simulink model "BMS_BIL_Wrapper"  (R2025b)
settings: Solver=FixedStepAuto  StartTime=0.0  StopTime=10.0  RelTol=1e-3  EnableMultiTasking=on
InitFcn:
  | battery_init;
  | Full_Charge_Volt=4.2; % unit volts
  | Cutoff_Volt=3; % unit volts
  | Delta=.02;
  | ContactorTime=20;
  | ContactorTimeOut=100;
  | High_TempLim=333;
  | Low_TempLim=253;
  | Sensor_Fault_Treshold=.02;
  | CurrentTimeout=1;
  | Allowed_Delta=.04;
  | Bal_On_Time=30;
  | Bal_Off_Time=5;
  | BalNotAct_Time=10;
values from neighbouring files (symbols this model uses):
  ADC_Volt_Resolution = .000089    (= 8.9e-05)    [MCU.m]
  bonka_R0 = [ ... (first row only)    [battery_init.m]
  bonka_SOC = [0, 0.1, 0.2, 0.3, 0.4, 0.5, 0.6, 0.7, 0.8, 0.9, 1.0]    [battery_init.m]
  bonka_T = [263.15, 273.15, 298.15, 313.15, 328.15]    [battery_init.m]
  Capacity = 5.200    (= 5.2)    [MCU.m]
  Charge_Rate = 1    [battery_init.m]
  Discharge_Rate = -1    [battery_init.m]
  R_NTC = 10000    [MCU.m]
  R_Pullup = 10000    [MCU.m]
  R_Sense = .01    (= 0.01)    [MCU.m]
  V_Bat_Div_Res = .00133    (= 0.00133)    [MCU.m]
  V_ISENSE_Res = .00000133    (= 1.33e-06)    [MCU.m]
undefined symbols (not defined in the file or in its folder): DiscIntNeverNeededParam
libraries: simulink x58, stm32f4xxblockslib x1, stm32blockslib x1
(part 1 of 2)
settings Model: DataDictionary=Needed_Buses.sldd  STM32="{\"SPIControllerTransfer\":[{\"ID\":\"Executable_Sim:1\"},{\"ID\":\"BMS_HIL_Wrapper:1\"},{\"ID\":\"BMS_HIL_Wrapper:200\"},{\"ID\":\"BMS_HIL_Wrapper:349\"},{\"ID\":\"BMS_BIL_Wrapper:1\"}],\"DigitalPortWrite\":[{\"ID\":\"Executable_Sim:197\"},{\"ID\":\"Executable_Sim:198\"},{\"ID\":\"BMS_BIL_Wrapper:898\"}]}"  Creator=Odonata-KJ  LastModifiedBy=Odonata-KJ
settings OptimizationCC: DefaultParameterBehavior=Inlined  EnhancedBackFolding=on  PassReuseOutputArgsAs=Individual arguments  ZeroExternalMemoryAtStartup=off  ZeroInternalMemoryAtStartup=off  MaxStackSize=512  OptimizeBlockOrder=speed  DifferentSizesBufferReuse=on  OptimizationCustomize=off  EfficientTunableParamExpr=on
settings DebuggingCC: ParameterTunabilityLossMsg=error
settings HardwareCC: ProdBitPerPointer=32.0  ProdBitPerSizeT=32.0  ProdBitPerPtrDiffT=32.0  ProdLargestAtomicInteger=Long  ProdLargestAtomicFloat=Double  ProdWordSize=32.0  ProdLongLongMode=on  ProdHWDeviceType=ARM Compatible->ARM Cortex-M  TargetBitPerPointer=64.0  TargetBitPerSizeT=64.0  TargetBitPerPtrDiffT=64.0  TargetLongLongMode=on  TargetIntDivRoundTo=Zero  TargetEndianess=LittleEndian  TargetWordSize=64.0  TargetHWDeviceType=MATLAB Host  ProdEqTarget=off
settings SFSimCC: MATLABDynamicMemAlloc=off
settings RTWCC: SystemTargetFile=ert.tlc  HardwareBoard=STM32F4xx Based  TemplateMakefile=ert_default_tmf  Toolchain=GNU Tools for ARM Embedded Processors  BuildConfiguration=Faster Runs  Description=Embedded Coder
settings CodeAppCC: ForceParamTrailComments=on  IgnoreCustomStorageClasses=off  OperatorAnnotations=on  SimulinkDataObjDesc=on  SFDataObjDesc=on  InsertBlockDesc=on
settings ERTTargetCC: ExtModeTransport=3.0  ExtModeStaticAlloc=on  ExtModeStaticAllocSize=2048.0  ExtModeMexFile=ext_xcp  ExtModeIntrfLevel=Level2 - Open  TargetLangStandard=C99 (ISO)

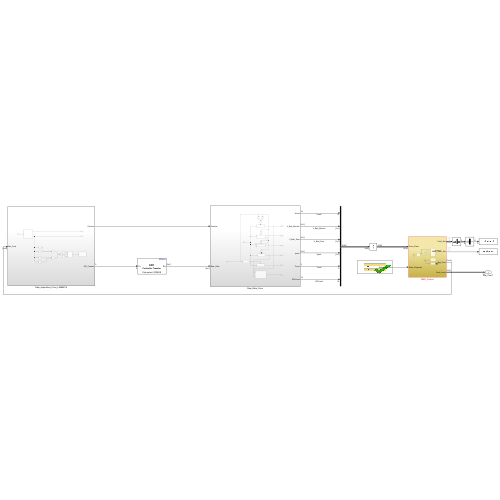
[thumbnail: Simulink's stored preview of the top-level diagram]
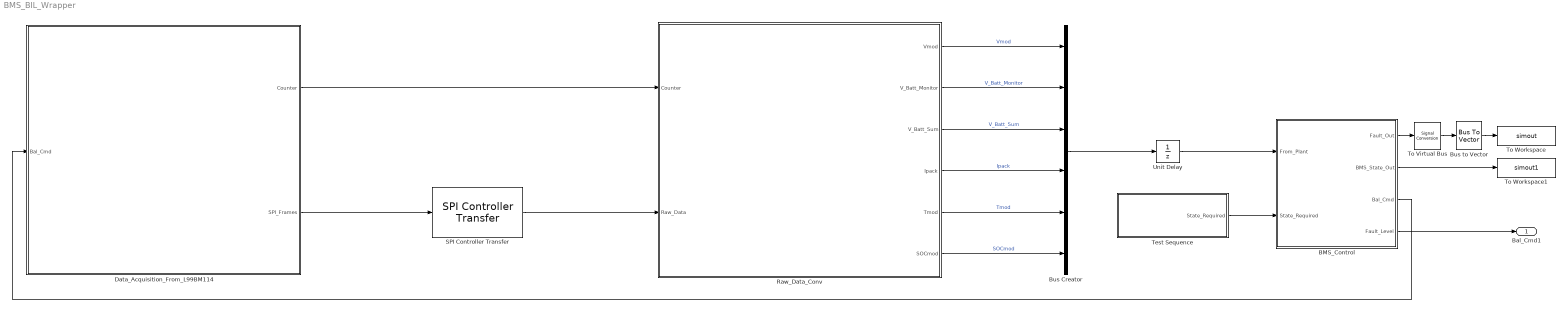
== system BMS_BIL_Wrapper ==
  BMS_Control : Subsystem
  Bus Creator : BusCreator  Inputs=6
  Bus to Vector : BusToVector
  Data_Acquisition_From_L99BM114 : Subsystem
  Raw_Data_Conv : Subsystem
  SPI Controller Transfer : stm32blockslib/SPI Controller Transfer  SPIModuleSelect=SPI1  ClockPolarity=Low  ClockPhase=1 Edge  SPIModule=uint32(0)  Mode=Master  BusSpeed=uint32(1000000)  FirstBitToTransfer=Most significant bit (MSB)  ClockMode=0  BlockFunction=Transfer  EnableRegisterAddress=on  RegisterAddress=0  OutputDataType=uint8  OutputDataLength=1  OutputStatus=off  BlockingMode=off  Timeout=0.001  DataBits=8  UseCustomSSPin=Provided by the SPI peripheral  ActiveLowSSPin=Active low  Port_Select=GPIOA  Pin=0
      settings: LibrarySourceBlock=stm32f4xxblockslib/SPI Controller Transfer
  Test Sequence : Test Sequence  TreatAsAtomicUnit=on
  To Virtual Bus : SignalConversion  ConversionOutput=Virtual bus  OverrideOpt=off
  To Workspace : ToWorkspace  VariableName=simout  SaveFormat=Structure With Time  SampleTime=-1
  To Workspace1 : ToWorkspace  VariableName=simout1  SaveFormat=Structure With Time  SampleTime=-1
  Unit Delay : UnitDelay  SampleTime=-1  HasFrameUpgradeWarning=on
  Bal_Cmd1 : Outport
  wires:
  Bus Creator/1 -> Unit Delay/1
  Test Sequence/1(State_Required) -> BMS_Control/2(State_Required)
  BMS_Control/1(Fault_Out) -> To Virtual Bus/1
  Data_Acquisition_From_L99BM114/2(SPI_Frames) -> SPI Controller Transfer/1
  SPI Controller Transfer/1 -> Raw_Data_Conv/2(Raw_Data)
  Raw_Data_Conv/1(Vmod) -> Bus Creator/1  "Vmod"
  Raw_Data_Conv/2(V_Batt_Monitor) -> Bus Creator/2  "V_Batt_Monitor"
  Raw_Data_Conv/3(V_Batt_Sum) -> Bus Creator/3  "V_Batt_Sum"
  Raw_Data_Conv/4(Ipack) -> Bus Creator/4  "Ipack"
  Raw_Data_Conv/5(Tmod) -> Bus Creator/5  "Tmod"
  Raw_Data_Conv/6(SOCmod) -> Bus Creator/6  "SOCmod"
  Data_Acquisition_From_L99BM114/1(Counter) -> Raw_Data_Conv/1(Counter)
  BMS_Control/2(BMS_State_Out) -> To Workspace1/1
  Bus to Vector/1 -> To Workspace/1
  To Virtual Bus/1 -> Bus to Vector/1
  BMS_Control/4(Fault_Level) -> Bal_Cmd1/1
  BMS_Control/3(Bal_Cmd) -> Data_Acquisition_From_L99BM114/1(Bal_Cmd)
  Unit Delay/1 -> BMS_Control/1(From_Plant)

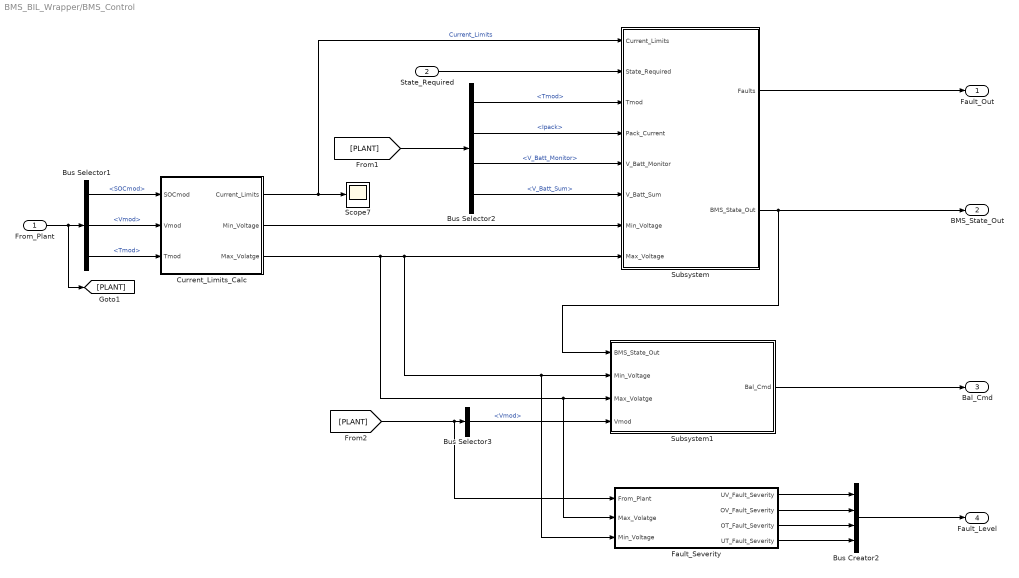
== system BMS_BIL_Wrapper/BMS_Control ==
  From_Plant : Inport
  State_Required : Inport  Port=2
  Bus Creator2 : BusCreator  Inputs=4
  Bus Selector1 : BusSelector  OutputSignals=SOCmod,Vmod,Tmod
  Bus Selector2 : BusSelector  OutputSignals=Tmod,Ipack,V_Batt_Monitor,V_Batt_Sum
  Bus Selector3 : BusSelector  OutputSignals=Vmod
  Current_Limits_Calc : Subsystem
  Fault_Severity : Subsystem
  Scope7 : Scope
      settings: ActiveDisplayYMinimum=-204.94239490667829  ActiveDisplayYMaximum=69.203108892530651  DataLoggingVariableName=ScopeData14
  Subsystem : Subsystem
  Subsystem1 : Subsystem
  Fault_Out : Outport
  BMS_State_Out : Outport  Port=2
  Bal_Cmd : Outport  Port=3
  Fault_Level : Outport  Port=4
  wires:
  Subsystem/2(BMS_State_Out) -> Subsystem1/1(BMS_State_Out), BMS_State_Out/1
  Subsystem/1(Faults) -> Fault_Out/1
  [PLANT] -> Bus Selector2/1
  State_Required/1 -> Subsystem/2(State_Required)
  Current_Limits_Calc/1(Current_Limits) -> Scope7/1, Subsystem/1(Current_Limits)  "Current_Limits"
  Current_Limits_Calc/3(Max_Volatge) -> Fault_Severity/2(Max_Volatge), Subsystem1/3(Max_Volatge), Fault_Severity/3(Min_Voltage), Subsystem1/2(Min_Voltage), Subsystem/8(Max_Voltage)
  Current_Limits_Calc/2(Min_Voltage) -> Subsystem/7(Min_Voltage)
  From_Plant/1 -> Bus Selector1/1, [PLANT]
  Bus Selector2/1 -> Subsystem/3(Tmod)  "<Tmod>"
  Bus Selector2/3 -> Subsystem/5(V_Batt_Monitor)  "<V_Batt_Monitor>"
  Bus Selector2/4 -> Subsystem/6(V_Batt_Sum)  "<V_Batt_Sum>"
  Bus Selector1/1 -> Current_Limits_Calc/1(SOCmod)  "<SOCmod>"
  Bus Selector1/2 -> Current_Limits_Calc/2(Vmod)  "<Vmod>"
  Bus Selector1/3 -> Current_Limits_Calc/3(Tmod)  "<Tmod>"
  Bus Selector2/2 -> Subsystem/4(Pack_Current)  "<Ipack>"
  Fault_Severity/4(UT_Fault_Severity) -> Bus Creator2/4
  Fault_Severity/1(UV_Fault_Severity) -> Bus Creator2/1
  Fault_Severity/2(OV_Fault_Severity) -> Bus Creator2/2
  Fault_Severity/3(OT_Fault_Severity) -> Bus Creator2/3
  [PLANT] -> Fault_Severity/1(From_Plant), Bus Selector3/1
  Bus Selector3/1 -> Subsystem1/4(Vmod)  "<Vmod>"
  Subsystem1/1(Bal_Cmd) -> Bal_Cmd/1
  Bus Creator2/1 -> Fault_Level/1

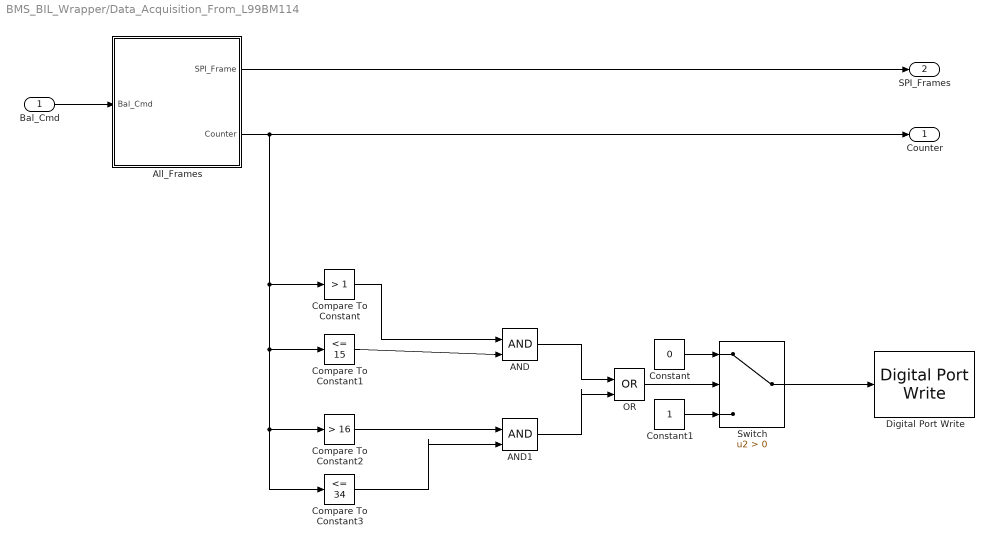
== system BMS_BIL_Wrapper/Data_Acquisition_From_L99BM114 ==
  Bal_Cmd : Inport
  AND : Logic  IconShape=distinctive  AllPortsSameDT=off  OutDataTypeStr=boolean
  AND1 : Logic  IconShape=distinctive  AllPortsSameDT=off  OutDataTypeStr=boolean
  All_Frames : Subsystem
  Compare To Constant : simulink/Logic and Bit Operations/Compare To Constant  relop=>  const=1  OutDataTypeStr=boolean
  Compare To Constant1 : simulink/Logic and Bit Operations/Compare To Constant  relop=<=  const=15  OutDataTypeStr=boolean
  Compare To Constant2 : simulink/Logic and Bit Operations/Compare To Constant  relop=>  const=16  OutDataTypeStr=boolean
  Compare To Constant3 : simulink/Logic and Bit Operations/Compare To Constant  relop=<=  const=34  OutDataTypeStr=boolean
  Constant : Constant  Value=0
  Constant1 : Constant
  Digital Port Write : stm32f4xxblockslib/Digital Port Write  PortName=GPIOB  PinNumber=[0]  ReadOperation=off  IOAsArray=on  EnableSimPort=off  hoistedMaskSrc=ECSoC/ECSimCodegen/Digital Port Write
  OR : Logic  Operator=OR  IconShape=distinctive  AllPortsSameDT=off  OutDataTypeStr=boolean
  Switch : Switch  Criteria=u2 > Threshold  SaturateOnIntegerOverflow=off  InputSameDT=off
  Counter : Outport
  SPI_Frames : Outport  Port=2
  wires:
  All_Frames/2(Counter) -> Compare To Constant2/1, Compare To Constant3/1, Compare To Constant1/1, Compare To Constant/1, Counter/1
  All_Frames/1(SPI_Frame) -> SPI_Frames/1
  Bal_Cmd/1 -> All_Frames/1(Bal_Cmd)
  Compare To Constant/1 -> AND/1
  Compare To Constant1/1 -> AND/2
  AND/1 -> OR/1
  Compare To Constant2/1 -> AND1/1
  Compare To Constant3/1 -> AND1/2
  AND1/1 -> OR/2
  OR/1 -> Switch/2
  Constant/1 -> Switch/1
  Constant1/1 -> Switch/3
  Switch/1 -> Digital Port Write/1

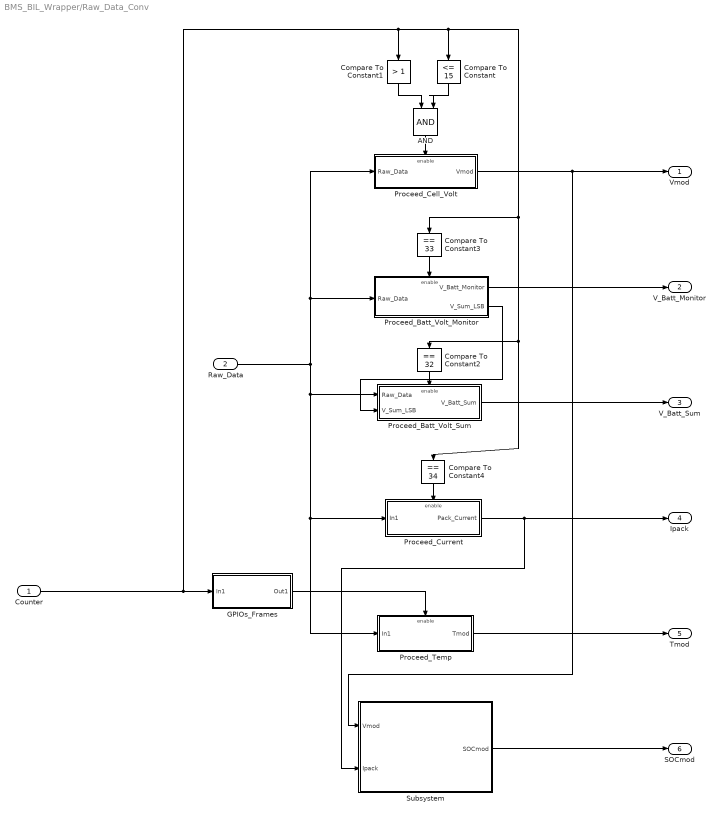
== system BMS_BIL_Wrapper/Raw_Data_Conv ==
  Counter : Inport
  Raw_Data : Inport  Port=2
  AND : Logic  IconShape=distinctive  AllPortsSameDT=off  OutDataTypeStr=boolean
  Compare To Constant : simulink/Logic and Bit Operations/Compare To Constant  relop=<=  const=15  OutDataTypeStr=boolean
  Compare To Constant1 : simulink/Logic and Bit Operations/Compare To Constant  relop=>  const=1  OutDataTypeStr=boolean
  Compare To Constant2 : simulink/Logic and Bit Operations/Compare To Constant  relop===  const=32  OutDataTypeStr=boolean
  Compare To Constant3 : simulink/Logic and Bit Operations/Compare To Constant  relop===  const=33  OutDataTypeStr=boolean
  Compare To Constant4 : simulink/Logic and Bit Operations/Compare To Constant  relop===  const=34  OutDataTypeStr=boolean
  GPIOs_Frames : Subsystem
  Proceed_Batt_Volt_Monitor : Subsystem  TreatAsAtomicUnit=on
  Proceed_Batt_Volt_Sum : Subsystem  TreatAsAtomicUnit=on
  Proceed_Cell_Volt : Subsystem  TreatAsAtomicUnit=on
  Proceed_Current : Subsystem
  Proceed_Temp : Subsystem
  Subsystem : Subsystem
  Vmod : Outport
  V_Batt_Monitor : Outport  Port=2
  V_Batt_Sum : Outport  Port=3
  Ipack : Outport  Port=4
  Tmod : Outport  Port=5
  SOCmod : Outport  Port=6
  wires:
  Proceed_Current/1(Pack_Current) -> Ipack/1, Subsystem/2(Ipack)
  Raw_Data/1 -> Proceed_Cell_Volt/1(Raw_Data), Proceed_Batt_Volt_Monitor/1(Raw_Data), Proceed_Temp/1(In1), Proceed_Current/1(In1), Proceed_Batt_Volt_Sum/1(Raw_Data)
  AND/1 -> Proceed_Cell_Volt/Enable
  Proceed_Batt_Volt_Monitor/2(V_Sum_LSB) -> Proceed_Batt_Volt_Sum/2(V_Sum_LSB)
  Proceed_Batt_Volt_Sum/1(V_Batt_Sum) -> V_Batt_Sum/1
  GPIOs_Frames/1(Out1) -> Proceed_Temp/Enable
  Counter/1 -> Compare To Constant3/1, Compare To Constant2/1, Compare To Constant4/1, Compare To Constant/1, Compare To Constant1/1, GPIOs_Frames/1(In1)
  Compare To Constant2/1 -> Proceed_Batt_Volt_Sum/Enable
  Compare To Constant1/1 -> AND/1
  Compare To Constant/1 -> AND/2
  Compare To Constant3/1 -> Proceed_Batt_Volt_Monitor/Enable
  Compare To Constant4/1 -> Proceed_Current/Enable
  Proceed_Temp/1(Tmod) -> Tmod/1
  Proceed_Cell_Volt/1(Vmod) -> Vmod/1, Subsystem/1(Vmod)
  Subsystem/1(SOCmod) -> SOCmod/1
  Proceed_Batt_Volt_Monitor/1(V_Batt_Monitor) -> V_Batt_Monitor/1

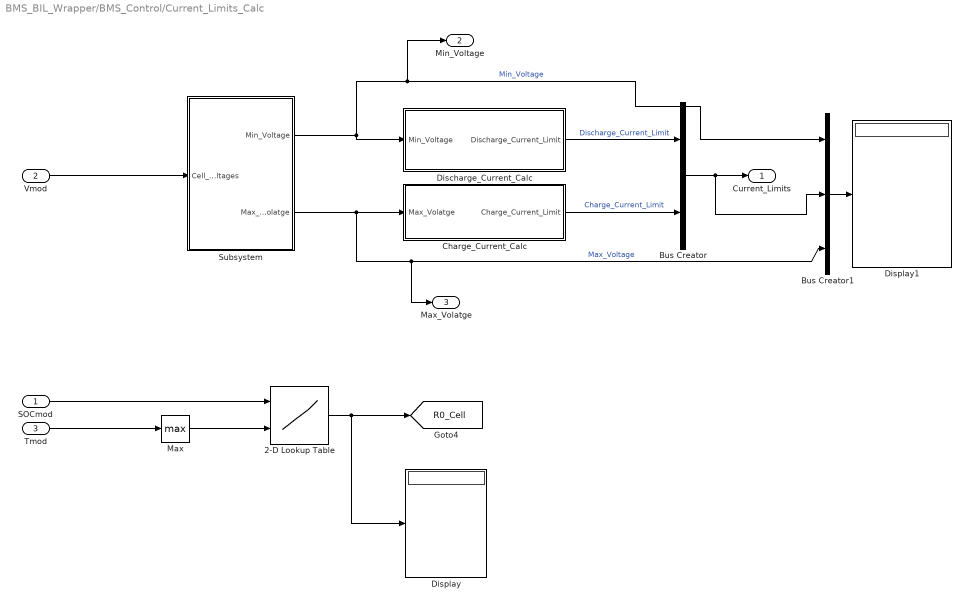
== system BMS_BIL_Wrapper/BMS_Control/Current_Limits_Calc ==
  SOCmod : Inport
  Vmod : Inport  Port=2
  Tmod : Inport  Port=3
  2-D Lookup Table : Lookup_n-D  BreakpointsForDimension1=bonka_SOC  BreakpointsForDimension2=bonka_T  Table=bonka_R0  InternalRulePriority=Speed  RndMeth=Simplest
      settings: InputPortMap=u0,u1
  Bus Creator : BusCreator  Inputs=2
  Bus Creator1 : BusCreator  Inputs=3
  Charge_Current_Calc : Subsystem
  Discharge_Current_Calc : Subsystem
  Display : Display
  Display1 : Display
  Max : MinMax  Function=max
  Subsystem : Subsystem
  Current_Limits : Outport
  Min_Voltage : Outport  Port=2
  Max_Volatge : Outport  Port=3
  tag scope: R0_Cell=global
  wires:
  Max/1 -> 2-D Lookup Table/2
  2-D Lookup Table/1 -> [R0_Cell], Display/1
  SOCmod/1 -> 2-D Lookup Table/1
  Bus Creator1/1 -> Display1/1
  Bus Creator/1 -> Current_Limits/1, Bus Creator1/2
  Charge_Current_Calc/1(Charge_Current_Limit) -> Bus Creator/2  "Charge_Current_Limit"
  Discharge_Current_Calc/1(Discharge_Current_Limit) -> Bus Creator/1  "Discharge_Current_Limit"
  Subsystem/2(Max_Volatge) -> Charge_Current_Calc/1(Max_Volatge), Max_Volatge/1, Bus Creator1/3  "Max_Voltage"
  Tmod/1 -> Max/1
  Subsystem/1(Min_Voltage) -> Min_Voltage/1, Bus Creator1/1, Discharge_Current_Calc/1(Min_Voltage)  "Min_Voltage"
  Vmod/1 -> Subsystem/1(Cell_Voltages)

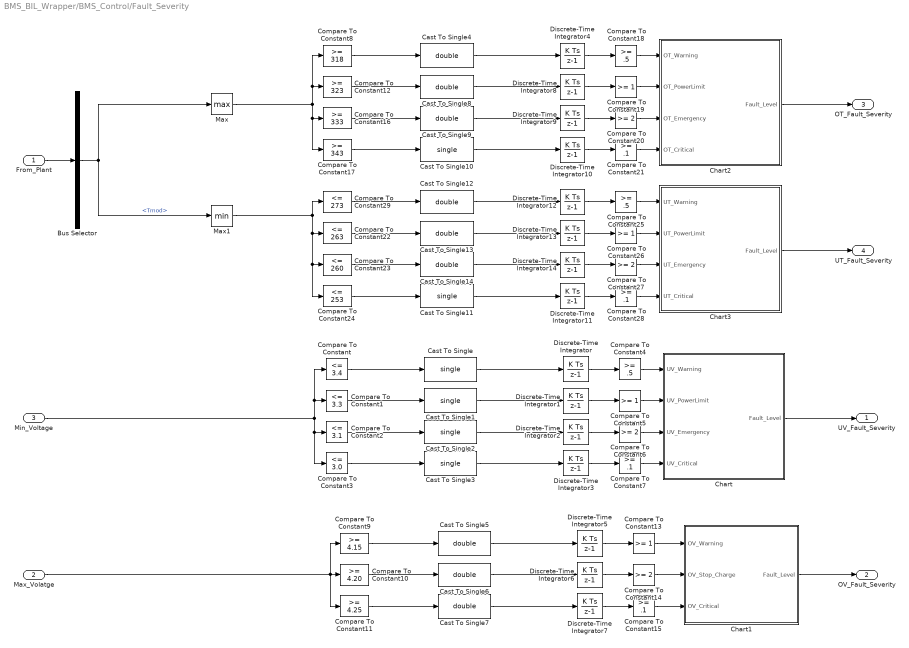
== system BMS_BIL_Wrapper/BMS_Control/Fault_Severity ==
  From_Plant : Inport
  Max_Volatge : Inport  Port=2
  Min_Voltage : Inport  Port=3
  Bus Selector : BusSelector  OutputSignals=Tmod
  Cast To Single{,1..3,10..11} (6 alike) : DataTypeConversion  OutDataTypeStr=single  SaturateOnIntegerOverflow=off  RndMeth=Floor
  Cast To Single{4..9,12..14} (9 alike) : DataTypeConversion  OutDataTypeStr=double  SaturateOnIntegerOverflow=off  RndMeth=Floor
  Chart : Stateflow chart  TreatAsAtomicUnit=on
  Chart1 : Stateflow chart  TreatAsAtomicUnit=on
  Chart2 : Stateflow chart  TreatAsAtomicUnit=on
  Chart3 : Stateflow chart  TreatAsAtomicUnit=on
  Compare To Constant : simulink/Logic and Bit Operations/Compare To Constant  relop=<=  const=3.4  OutDataTypeStr=boolean
  Compare To Constant1 : simulink/Logic and Bit Operations/Compare To Constant  relop=<=  const=3.3  OutDataTypeStr=boolean
  Compare To Constant10 : simulink/Logic and Bit Operations/Compare To Constant  relop=>=  const=4.20  OutDataTypeStr=boolean
  Compare To Constant11 : simulink/Logic and Bit Operations/Compare To Constant  relop=>=  const=4.25  OutDataTypeStr=boolean
  Compare To Constant12 : simulink/Logic and Bit Operations/Compare To Constant  relop=>=  const=323  OutDataTypeStr=boolean
  Compare To Constant{5,13,19,26} (4 alike) : simulink/Logic and Bit Operations/Compare To Constant  relop=>=  const=1  OutDataTypeStr=boolean
  Compare To Constant{6,14,20,27} (4 alike) : simulink/Logic and Bit Operations/Compare To Constant  relop=>=  const=2  OutDataTypeStr=boolean
  Compare To Constant{7,15,21,28} (4 alike) : simulink/Logic and Bit Operations/Compare To Constant  relop=>=  const=.1  OutDataTypeStr=boolean
  Compare To Constant16 : simulink/Logic and Bit Operations/Compare To Constant  relop=>=  const=333  OutDataTypeStr=boolean
  Compare To Constant17 : simulink/Logic and Bit Operations/Compare To Constant  relop=>=  const=343  OutDataTypeStr=boolean
  Compare To Constant18 : simulink/Logic and Bit Operations/Compare To Constant  relop=>=  const=.5  OutDataTypeStr=boolean
  Compare To Constant2 : simulink/Logic and Bit Operations/Compare To Constant  relop=<=  const=3.1  OutDataTypeStr=boolean
  Compare To Constant22 : simulink/Logic and Bit Operations/Compare To Constant  relop=<=  const=263  OutDataTypeStr=boolean
  Compare To Constant23 : simulink/Logic and Bit Operations/Compare To Constant  relop=<=  const=260  OutDataTypeStr=boolean
  Compare To Constant24 : simulink/Logic and Bit Operations/Compare To Constant  relop=<=  const=253  OutDataTypeStr=boolean
  Compare To Constant25 : simulink/Logic and Bit Operations/Compare To Constant  relop=>=  const=.5  OutDataTypeStr=boolean
  Compare To Constant29 : simulink/Logic and Bit Operations/Compare To Constant  relop=<=  const=273  OutDataTypeStr=boolean
  Compare To Constant3 : simulink/Logic and Bit Operations/Compare To Constant  relop=<=  const=3.0  OutDataTypeStr=boolean
  Compare To Constant4 : simulink/Logic and Bit Operations/Compare To Constant  relop=>=  const=.5  OutDataTypeStr=boolean
  Compare To Constant8 : simulink/Logic and Bit Operations/Compare To Constant  relop=>=  const=318  OutDataTypeStr=boolean
  Compare To Constant9 : simulink/Logic and Bit Operations/Compare To Constant  relop=>=  const=4.15  OutDataTypeStr=boolean
  Discrete-Time Integrator{,1..14} (15 alike) : DiscreteIntegrator  SampleTime=.001  ICPrevOutput=DiscIntNeverNeededParam  ICPrevScaledInput=DiscIntNeverNeededParam
  Max : MinMax  Function=max
  Max1 : MinMax
  UV_Fault_Severity : Outport
  OV_Fault_Severity : Outport  Port=2
  OT_Fault_Severity : Outport  Port=3
  UT_Fault_Severity : Outport  Port=4
  wires:
  From_Plant/1 -> Bus Selector/1
  Min_Voltage/1 -> Compare To Constant3/1, Compare To Constant2/1, Compare To Constant/1, Compare To Constant1/1
  Compare To Constant/1 -> Cast To Single/1
  Compare To Constant1/1 -> Cast To Single1/1
  Compare To Constant2/1 -> Cast To Single2/1
  Compare To Constant3/1 -> Cast To Single3/1
  Cast To Single/1 -> Discrete-Time Integrator/1
  Cast To Single1/1 -> Discrete-Time Integrator1/1
  Cast To Single2/1 -> Discrete-Time Integrator2/1
  Discrete-Time Integrator/1 -> Compare To Constant4/1
  Discrete-Time Integrator1/1 -> Compare To Constant5/1
  Discrete-Time Integrator2/1 -> Compare To Constant6/1
  Discrete-Time Integrator3/1 -> Compare To Constant7/1
  Cast To Single3/1 -> Discrete-Time Integrator3/1
  Compare To Constant4/1 -> Chart/1(UV_Warning)
  Compare To Constant5/1 -> Chart/2(UV_PowerLimit)
  Compare To Constant6/1 -> Chart/3(UV_Emergency)
  Compare To Constant7/1 -> Chart/4(UV_Critical)
  Chart/1(Fault_Level) -> UV_Fault_Severity/1
  Compare To Constant14/1 -> Chart1/2(OV_Stop_Charge)
  Max_Volatge/1 -> Compare To Constant9/1, Compare To Constant11/1, Compare To Constant10/1
  Discrete-Time Integrator6/1 -> Compare To Constant14/1
  Discrete-Time Integrator5/1 -> Compare To Constant13/1
  Compare To Constant13/1 -> Chart1/1(OV_Warning)
  Cast To Single6/1 -> Discrete-Time Integrator6/1
  Cast To Single7/1 -> Discrete-Time Integrator7/1
  Compare To Constant10/1 -> Cast To Single6/1
  Compare To Constant9/1 -> Cast To Single5/1
  Compare To Constant15/1 -> Chart1/3(OV_Critical)
  Compare To Constant11/1 -> Cast To Single7/1
  Chart1/1(Fault_Level) -> OV_Fault_Severity/1
  Discrete-Time Integrator7/1 -> Compare To Constant15/1
  Cast To Single5/1 -> Discrete-Time Integrator5/1
  Bus Selector/1 -> Max/1, Max1/1  "<Tmod>"
  Discrete-Time Integrator4/1 -> Compare To Constant18/1
  Compare To Constant20/1 -> Chart2/3(OT_Emergency)
  Max/1 -> Compare To Constant8/1, Compare To Constant12/1, Compare To Constant17/1, Compare To Constant16/1
  Discrete-Time Integrator9/1 -> Compare To Constant20/1
  Discrete-Time Integrator8/1 -> Compare To Constant19/1
  Compare To Constant19/1 -> Chart2/2(OT_PowerLimit)
  Cast To Single9/1 -> Discrete-Time Integrator9/1
  Cast To Single10/1 -> Discrete-Time Integrator10/1
  Cast To Single4/1 -> Discrete-Time Integrator4/1
  Compare To Constant16/1 -> Cast To Single9/1
  Compare To Constant12/1 -> Cast To Single8/1
  Compare To Constant21/1 -> Chart2/4(OT_Critical)
  Compare To Constant8/1 -> Cast To Single4/1
  Compare To Constant18/1 -> Chart2/1(OT_Warning)
  Compare To Constant17/1 -> Cast To Single10/1
  Chart2/1(Fault_Level) -> OT_Fault_Severity/1
  Discrete-Time Integrator10/1 -> Compare To Constant21/1
  Cast To Single8/1 -> Discrete-Time Integrator8/1
  Compare To Constant25/1 -> Chart3/1(UT_Warning)
  Max1/1 -> Compare To Constant22/1, Compare To Constant23/1, Compare To Constant24/1, Compare To Constant29/1
  Chart3/1(Fault_Level) -> UT_Fault_Severity/1
  Compare To Constant24/1 -> Cast To Single11/1
  Compare To Constant22/1 -> Cast To Single13/1
  Cast To Single13/1 -> Discrete-Time Integrator13/1
  Compare To Constant29/1 -> Cast To Single12/1
  Discrete-Time Integrator11/1 -> Compare To Constant28/1
  Compare To Constant23/1 -> Cast To Single14/1
  Discrete-Time Integrator14/1 -> Compare To Constant27/1
  Cast To Single14/1 -> Discrete-Time Integrator14/1
  Compare To Constant26/1 -> Chart3/2(UT_PowerLimit)
  Compare To Constant28/1 -> Chart3/4(UT_Critical)
  Cast To Single12/1 -> Discrete-Time Integrator12/1
  Discrete-Time Integrator13/1 -> Compare To Constant26/1
  Discrete-Time Integrator12/1 -> Compare To Constant25/1
  Compare To Constant27/1 -> Chart3/3(UT_Emergency)
  Cast To Single11/1 -> Discrete-Time Integrator11/1

== system BMS_BIL_Wrapper/BMS_Control/Subsystem ==
  Current_Limits : Inport
  State_Required : Inport  Port=2
  Tmod : Inport  Port=3
  Pack_Current : Inport  Port=4  OutDataTypeStr=single
  V_Batt_Monitor : Inport  Port=5
  V_Batt_Sum : Inport  Port=6  OutDataTypeStr=single
  Min_Voltage : Inport  Port=7
  Max_Voltage : Inport  Port=8
  BMS_States : Stateflow chart  TreatAsAtomicUnit=on
      settings: PortSchema="{\"entries\":[{\"content\":{\"sides\":[{\"content\":{\"connectorIds\":[\"In1\",\"In5\",\"In2\",\"In3\",\"In6\",\"In7\",\"In4\",\"In8\"]},\"type\":\"ConnectorPlacement.EquallySpacedRectSide\",\"uuid\":\"75752650-a65f-4df2-8429-36d8f2b8ac99\"},{\"content\":{\"connectorIds\":[\"Out1\",\"Out2\"],\"side\":\"RIGHT\"},\"type\":\"ConnectorPlacement.EquallySpacedRectSide\",\"uuid\":\"5c64a1aa-fdb2-4c0c-b2ff-5c47ddc01ea2\"},{\"content\":{\"side\":\"TOP\"},\"type\":\"ConnectorPlacement.EquallySpacedRectSide\",\"uuid\":\"c92e07e0-a1c3-44d4-87a0-5a0cb4ce56f3\"}]},\"type\":\"ConnectorPlacement.EquallySpacedConnector\",\"uuid\":\"9d97857d-a16c-4ff3-995b-4c10703be4f7\"}],\"packageUris\":[\"http://schema.mathworks.com/mf0/Connector/R2020b\"],\"version\":\"1.0\"}"
  Faults : Outport
  BMS_State_Out : Outport  Port=2
  wires:
  BMS_States/2(BMS_State_Out) -> BMS_State_Out/1
  BMS_States/1(Fault_out) -> Faults/1
  Current_Limits/1 -> BMS_States/1(Current_Limits)
  State_Required/1 -> BMS_States/5(State_Required)
  Min_Voltage/1 -> BMS_States/7(Min_Voltage)
  Max_Voltage/1 -> BMS_States/6(Max_Voltage)
  V_Batt_Sum/1 -> BMS_States/4(V_Batt_Sum)
  Pack_Current/1 -> BMS_States/3(Pack_Current)
  Tmod/1 -> BMS_States/2(Tmod)
  V_Batt_Monitor/1 -> BMS_States/8(V_Batt_Monitor)

== system BMS_BIL_Wrapper/BMS_Control/Subsystem1 ==
  BMS_State_Out : Inport
  Min_Voltage : Inport  Port=2
  Max_Volatge : Inport  Port=3
  Vmod : Inport  Port=4
  Chart : Stateflow chart  TreatAsAtomicUnit=on
  Bal_Cmd : Outport
  wires:
  BMS_State_Out/1 -> Chart/1(BMS_State_Out)
  Min_Voltage/1 -> Chart/2(Min_Voltage)
  Chart/1(Bal_Cmd) -> Bal_Cmd/1
  Vmod/1 -> Chart/4(Vmod)
  Max_Volatge/1 -> Chart/3(Max_Voltage)

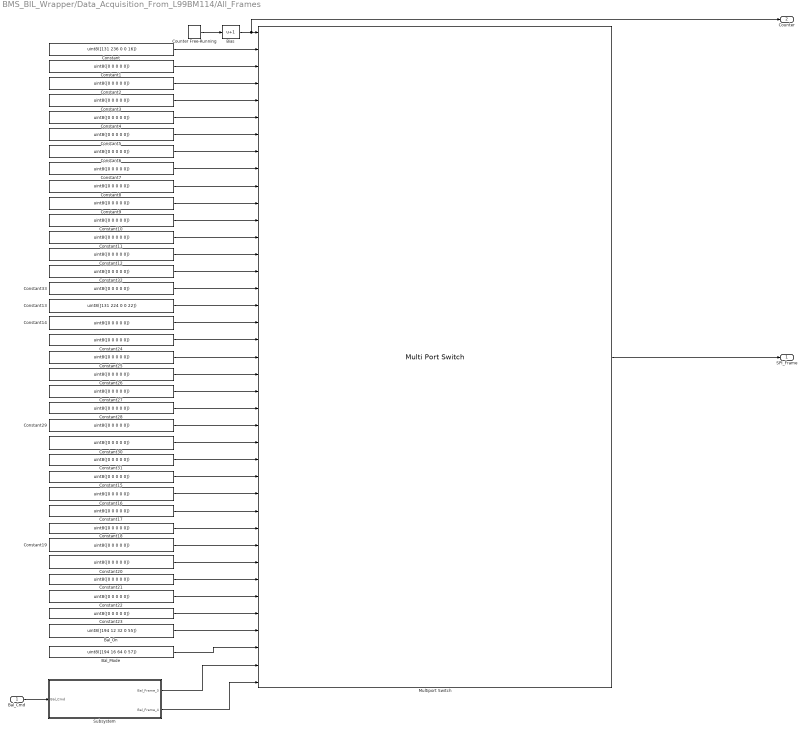
== system BMS_BIL_Wrapper/Data_Acquisition_From_L99BM114/All_Frames ==
  Bal_Cmd : Inport
  Bal_Mode : Constant  Value=uint8([194 16 64 0 57])
  Bal_On : Constant  Value=uint8([194 12 32 0 55])
  Bias : Bias  Bias=1  SaturateOnIntegerOverflow=off
  Constant : Constant  Value=uint8([131 236 0 0 16])
  Constant{1..12,14..33} (32 alike) : Constant  Value=uint8([0 0 0 0 0])
  Constant13 : Constant  Value=uint8([131 224 0 0 22])
  Counter Free-Running : simulink/Sources/Counter Free-Running  NumBits=16  tsamp=.001
  Multiport Switch : MultiPortSwitch  Inputs=38  OutDataTypeStr=uint8  SaturateOnIntegerOverflow=off  InputSameDT=off
  Subsystem : Subsystem
  SPI_Frame : Outport
  Counter : Outport  Port=2
  wires:
  Multiport Switch/1 -> SPI_Frame/1
  Counter Free-Running/1 -> Bias/1
  Bal_Cmd/1 -> Subsystem/1(Bal_Cmd)
  Bias/1 -> Multiport Switch/1, Counter/1
  Constant/1 -> Multiport Switch/2
  Constant1/1 -> Multiport Switch/3
  Constant2/1 -> Multiport Switch/4
  Constant3/1 -> Multiport Switch/5
  Constant4/1 -> Multiport Switch/6
  Constant5/1 -> Multiport Switch/7
  Constant6/1 -> Multiport Switch/8
  Constant7/1 -> Multiport Switch/9
  Constant8/1 -> Multiport Switch/10
  Constant9/1 -> Multiport Switch/11
  Constant10/1 -> Multiport Switch/12
  Constant11/1 -> Multiport Switch/13
  Constant12/1 -> Multiport Switch/14
  Constant33/1 -> Multiport Switch/16
  Constant32/1 -> Multiport Switch/15
  Constant13/1 -> Multiport Switch/17
  Constant14/1 -> Multiport Switch/18
  Constant24/1 -> Multiport Switch/19
  Constant25/1 -> Multiport Switch/20
  Constant26/1 -> Multiport Switch/21
  Constant27/1 -> Multiport Switch/22
  Constant28/1 -> Multiport Switch/23
  Constant29/1 -> Multiport Switch/24
  Constant31/1 -> Multiport Switch/26
  Constant30/1 -> Multiport Switch/25
  Constant15/1 -> Multiport Switch/27
  Constant16/1 -> Multiport Switch/28
  Constant17/1 -> Multiport Switch/29
  Constant18/1 -> Multiport Switch/30
  Constant19/1 -> Multiport Switch/31
  Constant20/1 -> Multiport Switch/32
  Constant21/1 -> Multiport Switch/33
  Constant22/1 -> Multiport Switch/34
  Constant23/1 -> Multiport Switch/35
  Subsystem/2(Bal_Frame_4) -> Multiport Switch/39
  Subsystem/1(Bal_Frame_3) -> Multiport Switch/38
  Bal_Mode/1 -> Multiport Switch/37
  Bal_On/1 -> Multiport Switch/36

== system BMS_BIL_Wrapper/Raw_Data_Conv/GPIOs_Frames ==
  In1 : Inport
  Compare To Constant : simulink/Logic and Bit Operations/Compare To Constant  relop===  const=7  OutDataTypeStr=boolean
  Compare To Constant1 : simulink/Logic and Bit Operations/Compare To Constant  relop===  const=8  OutDataTypeStr=boolean
  Compare To Constant2 : simulink/Logic and Bit Operations/Compare To Constant  relop===  const=9  OutDataTypeStr=boolean
  Compare To Constant3 : simulink/Logic and Bit Operations/Compare To Constant  relop===  const=10  OutDataTypeStr=boolean
  Compare To Constant4 : simulink/Logic and Bit Operations/Compare To Constant  relop===  const=13  OutDataTypeStr=boolean
  OR : Logic  Operator=OR  Inputs=5  IconShape=distinctive  AllPortsSameDT=off  OutDataTypeStr=boolean
  Out1 : Outport
  wires:
  Compare To Constant2/1 -> OR/3
  Compare To Constant1/1 -> OR/2
  Compare To Constant/1 -> OR/1
  Compare To Constant3/1 -> OR/4
  Compare To Constant4/1 -> OR/5
  In1/1 -> Compare To Constant2/1, Compare To Constant3/1, Compare To Constant4/1, Compare To Constant1/1, Compare To Constant/1
  OR/1 -> Out1/1

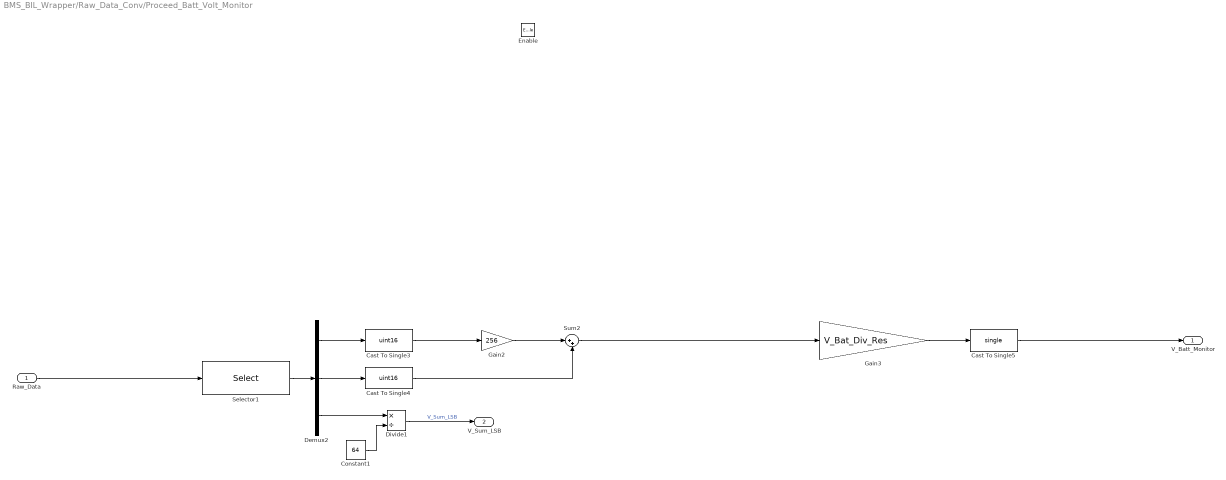
== system BMS_BIL_Wrapper/Raw_Data_Conv/Proceed_Batt_Volt_Monitor ==
  Raw_Data : Inport
  Enable : EnablePort
  Cast To Single3 : DataTypeConversion  OutDataTypeStr=uint16  SaturateOnIntegerOverflow=off  RndMeth=Floor
  Cast To Single4 : DataTypeConversion  OutDataTypeStr=uint16  SaturateOnIntegerOverflow=off  RndMeth=Floor
  Cast To Single5 : DataTypeConversion  OutDataTypeStr=single  SaturateOnIntegerOverflow=off  RndMeth=Floor
  Constant1 : Constant  Value=64
  Demux2 : Demux  Outputs=3
  Divide1 : Product  Inputs=*/
  Gain2 : Gain  Gain=256
  Gain3 : Gain  Gain=V_Bat_Div_Res
  Selector1 : Selector  InputPortWidth=5  IndexOptions=Index vector (dialog)  Indices=[3:5]  OutputSizes=1
  Sum2 : Sum  Inputs=|++
  V_Batt_Monitor : Outport
  V_Sum_LSB : Outport  Port=2
  wires:
  Raw_Data/1 -> Selector1/1
  Selector1/1 -> Demux2/1
  Demux2/1 -> Cast To Single3/1
  Demux2/2 -> Cast To Single4/1
  Cast To Single3/1 -> Gain2/1
  Gain2/1 -> Sum2/1
  Cast To Single4/1 -> Sum2/2
  Demux2/3 -> Divide1/1
  Constant1/1 -> Divide1/2
  Sum2/1 -> Gain3/1
  Gain3/1 -> Cast To Single5/1
  Cast To Single5/1 -> V_Batt_Monitor/1
  Divide1/1 -> V_Sum_LSB/1  "V_Sum_LSB"

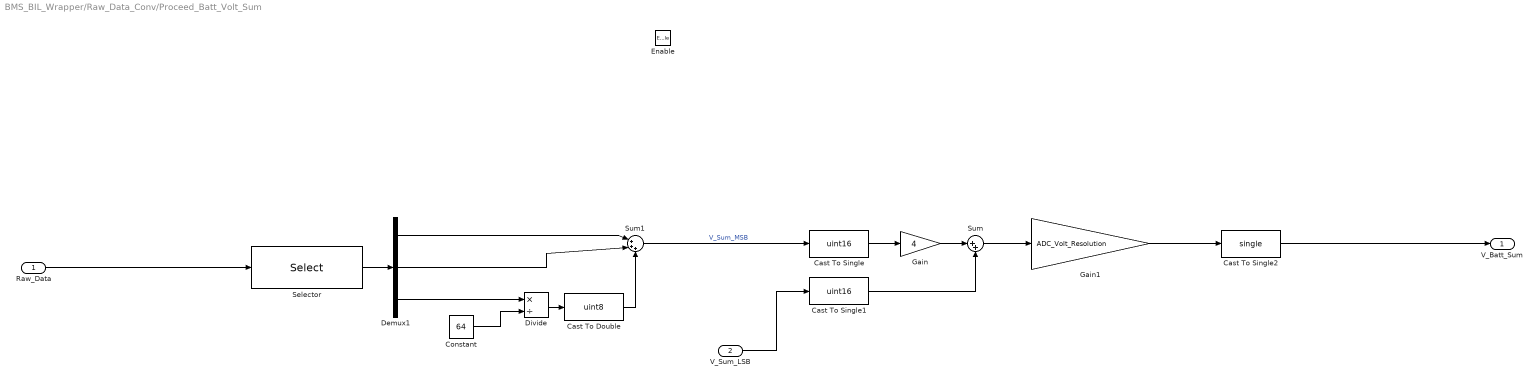
== system BMS_BIL_Wrapper/Raw_Data_Conv/Proceed_Batt_Volt_Sum ==
  Raw_Data : Inport
  V_Sum_LSB : Inport  Port=2
  Enable : EnablePort
  Cast To Double : DataTypeConversion  OutDataTypeStr=uint8  SaturateOnIntegerOverflow=off  RndMeth=Floor
  Cast To Single : DataTypeConversion  OutDataTypeStr=uint16  SaturateOnIntegerOverflow=off  RndMeth=Floor
  Cast To Single1 : DataTypeConversion  OutDataTypeStr=uint16  SaturateOnIntegerOverflow=off  RndMeth=Floor
  Cast To Single2 : DataTypeConversion  OutDataTypeStr=single  SaturateOnIntegerOverflow=off  RndMeth=Floor
  Constant : Constant  Value=64
  Demux1 : Demux  Outputs=3
  Divide : Product  Inputs=*/
  Gain : Gain  Gain=4
  Gain1 : Gain  Gain=ADC_Volt_Resolution
  Selector : Selector  InputPortWidth=5  IndexOptions=Index vector (dialog)  Indices=[3:5]  OutputSizes=1
  Sum : Sum  Inputs=|++
  Sum1 : Sum  Inputs=|+++
  V_Batt_Sum : Outport
  wires:
  Gain1/1 -> Cast To Single2/1
  Raw_Data/1 -> Selector/1
  Gain/1 -> Sum/1
  Cast To Single1/1 -> Sum/2
  Sum/1 -> Gain1/1
  Cast To Single/1 -> Gain/1
  Cast To Single2/1 -> V_Batt_Sum/1
  Selector/1 -> Demux1/1
  Demux1/3 -> Divide/1
  Constant/1 -> Divide/2
  Demux1/1 -> Sum1/1
  Demux1/2 -> Sum1/2
  Divide/1 -> Cast To Double/1
  Cast To Double/1 -> Sum1/3
  Sum1/1 -> Cast To Single/1  "V_Sum_MSB"
  V_Sum_LSB/1 -> Cast To Single1/1

== system BMS_BIL_Wrapper/Raw_Data_Conv/Proceed_Cell_Volt ==
  Raw_Data : Inport
  Enable : EnablePort
  Cast To Single : DataTypeConversion  OutDataTypeStr=uint16  SaturateOnIntegerOverflow=off  RndMeth=Floor
  Cast To Single1 : DataTypeConversion  OutDataTypeStr=uint16  SaturateOnIntegerOverflow=off  RndMeth=Floor
  Cast To Single2 : DataTypeConversion  OutDataTypeStr=single  SaturateOnIntegerOverflow=off  RndMeth=Floor
  Demux : Demux  Outputs=2
  Gain : Gain  Gain=256
  Gain1 : Gain  Gain=ADC_Volt_Resolution
  Selector : Selector  InputPortWidth=5  IndexOptions=Index vector (dialog)  Indices=[3:4]  OutputSizes=1
  Sum : Sum  Inputs=|++
  Tapped Delay : simulink/Discrete/Tapped Delay  vinit=0  samptime=-1  NumDelays=14  DelayOrder=Oldest  includeCurrent=off
  Vmod : Outport
  wires:
  Gain1/1 -> Cast To Single2/1
  Demux/1 -> Cast To Single/1
  Raw_Data/1 -> Selector/1
  Gain/1 -> Sum/1
  Demux/2 -> Cast To Single1/1
  Selector/1 -> Demux/1
  Cast To Single1/1 -> Sum/2
  Sum/1 -> Gain1/1
  Cast To Single/1 -> Gain/1
  Cast To Single2/1 -> Tapped Delay/1
  Tapped Delay/1 -> Vmod/1

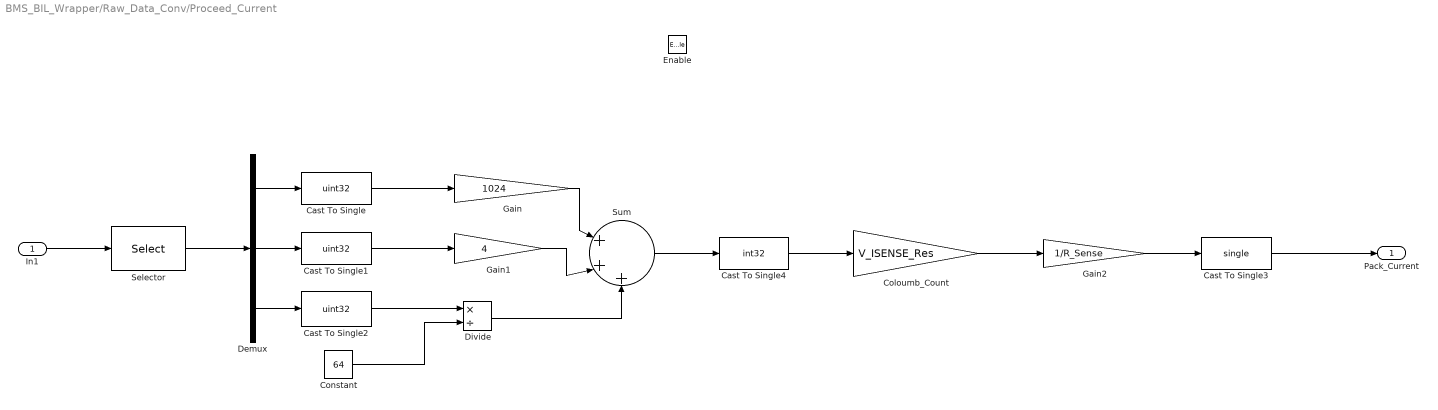
== system BMS_BIL_Wrapper/Raw_Data_Conv/Proceed_Current ==
  In1 : Inport
  Enable : EnablePort
  Cast To Single : DataTypeConversion  OutDataTypeStr=uint32  SaturateOnIntegerOverflow=off  RndMeth=Floor
  Cast To Single1 : DataTypeConversion  OutDataTypeStr=uint32  SaturateOnIntegerOverflow=off  RndMeth=Floor
  Cast To Single2 : DataTypeConversion  OutDataTypeStr=uint32  SaturateOnIntegerOverflow=off  RndMeth=Floor
  Cast To Single3 : DataTypeConversion  OutDataTypeStr=single  SaturateOnIntegerOverflow=off  RndMeth=Floor
  Cast To Single4 : DataTypeConversion  OutDataTypeStr=int32  SaturateOnIntegerOverflow=off  RndMeth=Floor
  Coloumb_Count : Gain  Gain=V_ISENSE_Res
  Constant : Constant  Value=64
  Demux : Demux  Outputs=3
  Divide : Product  Inputs=*/
  Gain : Gain  Gain=1024
  Gain1 : Gain  Gain=4
  Gain2 : Gain  Gain=1/R_Sense
  Selector : Selector  InputPortWidth=5  IndexOptions=Index vector (dialog)  Indices=[3:5]  OutputSizes=1
  Sum : Sum  Inputs=|+++
  Pack_Current : Outport
  wires:
  In1/1 -> Selector/1
  Selector/1 -> Demux/1
  Demux/1 -> Cast To Single/1
  Demux/2 -> Cast To Single1/1
  Demux/3 -> Cast To Single2/1
  Cast To Single/1 -> Gain/1
  Cast To Single1/1 -> Gain1/1
  Cast To Single2/1 -> Divide/1
  Sum/1 -> Cast To Single4/1
  Gain/1 -> Sum/1
  Gain1/1 -> Sum/2
  Divide/1 -> Sum/3
  Cast To Single4/1 -> Coloumb_Count/1
  Coloumb_Count/1 -> Gain2/1
  Constant/1 -> Divide/2
  Cast To Single3/1 -> Pack_Current/1
  Gain2/1 -> Cast To Single3/1

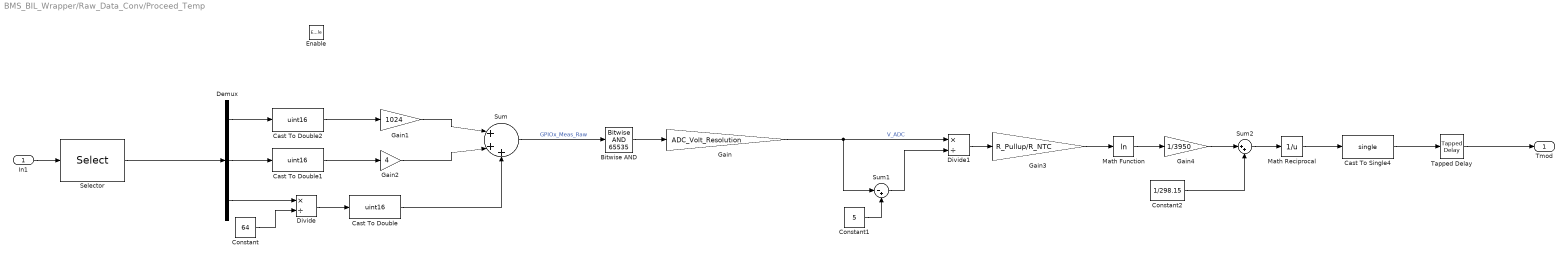
== system BMS_BIL_Wrapper/Raw_Data_Conv/Proceed_Temp ==
  In1 : Inport
  Enable : EnablePort
  Bitwise AND : simulink/Logic and Bit Operations/Bitwise Operator  logicop=AND  UseBitMask=on  BitMask=65535  BitMaskRealWorld=Stored Integer
      settings: LibrarySourceBlock=|
      | simulink/Quick Insert/Logic and Bit
      | Operations/Bitwise AND
  Cast To Double : DataTypeConversion  OutDataTypeStr=uint16  SaturateOnIntegerOverflow=off  RndMeth=Floor
  Cast To Double1 : DataTypeConversion  OutDataTypeStr=uint16  SaturateOnIntegerOverflow=off  RndMeth=Floor
  Cast To Double2 : DataTypeConversion  OutDataTypeStr=uint16  SaturateOnIntegerOverflow=off  RndMeth=Floor
  Cast To Single4 : DataTypeConversion  OutDataTypeStr=single  SaturateOnIntegerOverflow=off  RndMeth=Floor
  Constant : Constant  Value=64
  Constant1 : Constant  Value=5
  Constant2 : Constant  Value=1/298.15
  Demux : Demux  Outputs=3
  Divide : Product  Inputs=*/
  Divide1 : Product  Inputs=*/
  Gain : Gain  Gain=ADC_Volt_Resolution
  Gain1 : Gain  Gain=1024
  Gain2 : Gain  Gain=4
  Gain3 : Gain  Gain=R_Pullup/R_NTC
  Gain4 : Gain  Gain=1/3950
  Math Function : Math  Operator=log
  Math Reciprocal : Math  Operator=reciprocal  SignedPower=on
  Selector : Selector  InputPortWidth=5  IndexOptions=Index vector (dialog)  Indices=[3:5]  OutputSizes=1
  Sum : Sum  Inputs=|+++
  Sum1 : Sum  Inputs=|-+
  Sum2 : Sum  Inputs=|++
  Tapped Delay : simulink/Discrete/Tapped Delay  vinit=0.0  samptime=-1  NumDelays=5  DelayOrder=Oldest  includeCurrent=off
  Tmod : Outport
  wires:
  In1/1 -> Selector/1
  Selector/1 -> Demux/1
  Demux/3 -> Divide/1
  Constant/1 -> Divide/2
  Divide/1 -> Cast To Double/1
  Demux/2 -> Cast To Double1/1
  Demux/1 -> Cast To Double2/1
  Cast To Double2/1 -> Gain1/1
  Cast To Double1/1 -> Gain2/1
  Gain1/1 -> Sum/1
  Gain2/1 -> Sum/2
  Cast To Double/1 -> Sum/3
  Sum/1 -> Bitwise AND/1  "GPIOx_Meas_Raw"
  Bitwise AND/1 -> Gain/1
  Math Function/1 -> Gain4/1
  Gain3/1 -> Math Function/1
  Constant1/1 -> Sum1/2
  Sum1/1 -> Divide1/2
  Gain/1 -> Sum1/1, Divide1/1  "V_ADC"
  Gain4/1 -> Sum2/1
  Divide1/1 -> Gain3/1
  Constant2/1 -> Sum2/2
  Cast To Single4/1 -> Tapped Delay/1
  Math Reciprocal/1 -> Cast To Single4/1
  Sum2/1 -> Math Reciprocal/1
  Tapped Delay/1 -> Tmod/1

== system BMS_BIL_Wrapper/Raw_Data_Conv/Subsystem ==
  Vmod : Inport
  Ipack : Inport  Port=2
  1-D Lookup Table : Lookup_n-D  NumberOfTableDimensions=1  BreakpointsForDimension1=[3.0, 3.4, 3.6, 3.7, 3.8, 3.9, 4.0, 4.1, 4.2]  Table=[0.0, 0.1, 0.25, 0.45, 0.62, 0.78, 0.88, 0.95, 1.0]  InternalRulePriority=Speed  RndMeth=Simplest
  Cast To Double : DataTypeConversion  OutDataTypeStr=double  SaturateOnIntegerOverflow=off  RndMeth=Floor
  Cast To Single : DataTypeConversion  OutDataTypeStr=single  SaturateOnIntegerOverflow=off  RndMeth=Floor
  Discrete-Time Integrator : DiscreteIntegrator  SampleTime=-1  ICPrevOutput=DiscIntNeverNeededParam  ICPrevScaledInput=DiscIntNeverNeededParam
  Gain : Gain  Gain=1/(Capacity*3600)
  Sum : Sum  Inputs=|-+
  SOCmod : Outport
  wires:
  Ipack/1 -> Cast To Double/1
  Discrete-Time Integrator/1 -> Cast To Single/1
  Gain/1 -> Sum/1
  Vmod/1 -> 1-D Lookup Table/1
  1-D Lookup Table/1 -> Sum/2
  Sum/1 -> SOCmod/1
  Cast To Double/1 -> Discrete-Time Integrator/1
  Cast To Single/1 -> Gain/1

== system BMS_BIL_Wrapper/BMS_Control/Current_Limits_Calc/Charge_Current_Calc ==
  Max_Volatge : Inport
  " " : Gain  Gain=Charge_Rate
  Cast To Single : DataTypeConversion  OutDataTypeStr=single  SaturateOnIntegerOverflow=off  RndMeth=Floor
  Constant : Constant  Value=Full_Charge_Volt
  Divide : Product  Inputs=*/
  Max : MinMax  Function=max
  Sum : Sum  Inputs=|+-
  Charge_Current_Limit : Outport
  wires:
  Max/1 -> Divide/2
  " "/1 -> Cast To Single/1
  Cast To Single/1 -> Charge_Current_Limit/1
  Divide/1 -> " "/1
  [R0_Cell] -> Max/1
  Sum/1 -> Divide/1
  Max_Volatge/1 -> Sum/2
  Constant/1 -> Sum/1

== system BMS_BIL_Wrapper/BMS_Control/Current_Limits_Calc/Discharge_Current_Calc ==
  Min_Voltage : Inport
  Cast To Single : DataTypeConversion  OutDataTypeStr=single  SaturateOnIntegerOverflow=off  RndMeth=Floor
  Cutoff_Volt : Constant  Value=Cutoff_Volt
  Divide : Product  Inputs=*/
  Gain : Gain  Gain=Discharge_Rate
  Max : MinMax  Function=max
  Sum : Sum  Inputs=|+-
  Discharge_Current_Limit : Outport
  wires:
  [R0_Cell] -> Max/1
  Gain/1 -> Cast To Single/1
  Cast To Single/1 -> Discharge_Current_Limit/1
  Divide/1 -> Gain/1
  Max/1 -> Divide/2
  Sum/1 -> Divide/1
  Cutoff_Volt/1 -> Sum/2
  Min_Voltage/1 -> Sum/1

== system BMS_BIL_Wrapper/BMS_Control/Current_Limits_Calc/Subsystem ==
  Cell_Voltages : Inport
  Max : MinMax  Function=max
  MinMax : MinMax
  Min_Voltage : Outport
  Max_Volatge : Outport  Port=2
  wires:
  Max/1 -> Max_Volatge/1
  MinMax/1 -> Min_Voltage/1
  Cell_Voltages/1 -> MinMax/1, Max/1

== system BMS_BIL_Wrapper/Data_Acquisition_From_L99BM114/All_Frames/Subsystem ==
  Bal_Cmd : Inport
  Data Type Conversion : DataTypeConversion  OutDataTypeStr=uint8  SaturateOnIntegerOverflow=off  RndMeth=Floor
  Data Type Conversion1 : DataTypeConversion  OutDataTypeStr=uint8  SaturateOnIntegerOverflow=off  RndMeth=Floor
  Subsystem : Subsystem
  Vector Concatenate : Concatenate  NumInputs=5
  Vector Concatenate1 : Concatenate  NumInputs=5
  Bal_Frame_3 : Outport  OutDataTypeStr=uint8
  Bal_Frame_4 : Outport  Port=2  OutDataTypeStr=uint8
  wires:
  Bal_Cmd/1 -> Subsystem/1(Bal_Cmd)
  Subsystem/1(BalCell14_7_Byte_1) -> Vector Concatenate/1
  Subsystem/2(BalCell14_7_Byte_2) -> Vector Concatenate/2
  Subsystem/3(BalCell14_7_Byte_3) -> Vector Concatenate/3
  Subsystem/4(BalCell14_7_Byte_4) -> Vector Concatenate/4
  Subsystem/5(BalCell14_7_Byte_5) -> Vector Concatenate/5
  Vector Concatenate/1 -> Data Type Conversion/1
  Vector Concatenate1/1 -> Data Type Conversion1/1
  Subsystem/6(BalCell6_1_Byte_1) -> Vector Concatenate1/1
  Subsystem/7(BalCell6_1_Byte_2) -> Vector Concatenate1/2
  Subsystem/8(BalCell6_1_Byte_3) -> Vector Concatenate1/3
  Subsystem/9(BalCell6_1_Byte_4) -> Vector Concatenate1/4
  Subsystem/10(BalCell6_1_Byte_5) -> Vector Concatenate1/5
  Data Type Conversion/1 -> Bal_Frame_3/1
  Data Type Conversion1/1 -> Bal_Frame_4/1

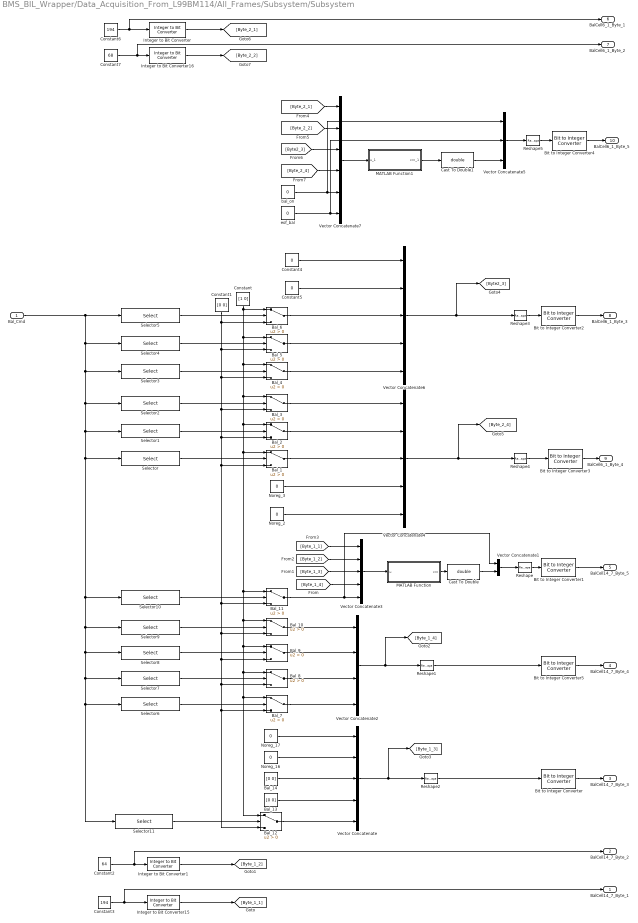
== system BMS_BIL_Wrapper/Data_Acquisition_From_L99BM114/All_Frames/Subsystem/Subsystem ==
  Bal_Cmd : Inport
  Bal_{1..12} (12 alike) : Switch  Criteria=u2 > Threshold  SaturateOnIntegerOverflow=off  InputSameDT=off
  Bal_13 : Constant  Value=[0 0]
  Bal_14 : Constant  Value=[0 0]
  Bit to Integer Converter{,1..5} (6 alike) : simulink/Logic and Bit Operations/Bit to Integer Converter  nbits=8  bitOrder=MSB first  signedOutputValues=Unsigned  outDtype=Inherit via internal rule  outDtypeSigned=Inherit via internal rule
  Cast To Double : DataTypeConversion  OutDataTypeStr=double  SaturateOnIntegerOverflow=off  RndMeth=Floor
  Cast To Double1 : DataTypeConversion  OutDataTypeStr=double  SaturateOnIntegerOverflow=off  RndMeth=Floor
  Constant : Constant  Value=[1 0]
  Constant1 : Constant  Value=[0 0]
  Constant2 : Constant  Value=64
  Constant3 : Constant  Value=194
  Constant4 : Constant  Value=0
  Constant5 : Constant  Value=0
  Constant6 : Constant  Value=194
  Constant7 : Constant  Value=68
  Integer to Bit Converter{,1,15..16} (4 alike) : simulink/Logic and Bit Operations/Integer to Bit Converter  nbits=8  signedInputValues=Unsigned  bitOrder=MSB first  outDtype=Inherit via internal rule
  MATLAB Function : MATLAB Function  TreatAsAtomicUnit=on
  MATLAB Function1 : MATLAB Function  TreatAsAtomicUnit=on
  Noreg_{2..3,16..17} (4 alike) : Constant  Value=0
  Reshape{,1..5} (6 alike) : Reshape  OutputDimensionality=Customize  OutputDimensions=[8,1]
  Selector : Selector  InputPortWidth=14  IndexOptions=Index vector (dialog)  Indices=1  OutputSizes=1
  Selector1 : Selector  InputPortWidth=14  IndexOptions=Index vector (dialog)  Indices=2  OutputSizes=1
  Selector10 : Selector  InputPortWidth=14  IndexOptions=Index vector (dialog)  Indices=11  OutputSizes=1
  Selector11 : Selector  InputPortWidth=14  IndexOptions=Index vector (dialog)  Indices=12  OutputSizes=1
  Selector2 : Selector  InputPortWidth=14  IndexOptions=Index vector (dialog)  Indices=3  OutputSizes=1
  Selector3 : Selector  InputPortWidth=14  IndexOptions=Index vector (dialog)  Indices=4  OutputSizes=1
  Selector4 : Selector  InputPortWidth=14  IndexOptions=Index vector (dialog)  Indices=5  OutputSizes=1
  Selector5 : Selector  InputPortWidth=14  IndexOptions=Index vector (dialog)  Indices=6  OutputSizes=1
  Selector6 : Selector  InputPortWidth=14  IndexOptions=Index vector (dialog)  Indices=7  OutputSizes=1
  Selector7 : Selector  InputPortWidth=14  IndexOptions=Index vector (dialog)  Indices=8  OutputSizes=1
  Selector8 : Selector  InputPortWidth=14  IndexOptions=Index vector (dialog)  Indices=9  OutputSizes=1
  Selector9 : Selector  InputPortWidth=14  IndexOptions=Index vector (dialog)  Indices=10  OutputSizes=1
  Vector Concatenate{,3..4,6} (4 alike) : Concatenate  NumInputs=5
  Vector Concatenate1 : Concatenate
  Vector Concatenate2 : Concatenate  NumInputs=4
  Vector Concatenate5 : Concatenate  NumInputs=3
  Vector Concatenate7 : Concatenate  NumInputs=6
  bal_on : Constant  Value=0
  eof_bal : Constant  Value=0
  BalCell14_7_Byte_1 : Outport
  BalCell14_7_Byte_2 : Outport  Port=2
  BalCell14_7_Byte_3 : Outport  Port=3
  BalCell14_7_Byte_4 : Outport  Port=4
  BalCell14_7_Byte_5 : Outport  Port=5
  BalCell6_1_Byte_1 : Outport  Port=6
  BalCell6_1_Byte_2 : Outport  Port=7
  BalCell6_1_Byte_3 : Outport  Port=8
  BalCell6_1_Byte_4 : Outport  Port=9
  BalCell6_1_Byte_5 : Outport  Port=10
  wires:
  Vector Concatenate5/1 -> Reshape5/1
  Cast To Double1/1 -> Vector Concatenate5/3
  Bal_6/1 -> Vector Concatenate6/3
  [Byte_1_3] -> Vector Concatenate3/3
  Bal_3/1 -> Vector Concatenate4/1
  [Byte_1_4] -> Vector Concatenate3/4
  [Byte2_3] -> Vector Concatenate7/3
  [Byte_2_1] -> Vector Concatenate7/1
  Bal_4/1 -> Vector Concatenate6/5
  Vector Concatenate1/1 -> Reshape/1
  Noreg_3/1 -> Vector Concatenate4/4
  Bal_12/1 -> Vector Concatenate/5
  Selector4/1 -> Bal_5/2
  Selector3/1 -> Bal_4/2
  Selector7/1 -> Bal_8/2
  Selector2/1 -> Bal_3/2
  Selector6/1 -> Bal_7/2
  Constant/1 -> Bal_12/1, Bal_7/1, Bal_8/1, Bal_9/1, Bal_10/1, Bal_11/1, Bal_1/1, Bal_2/1, Bal_3/1, Bal_4/1, Bal_5/1, Bal_6/1
  Selector1/1 -> Bal_2/2
  Bit to Integer Converter/1 -> BalCell14_7_Byte_3/1
  Integer to Bit Converter1/1 -> [Byte_1_2]
  Constant3/1 -> BalCell14_7_Byte_1/1, Integer to Bit Converter15/1
  Constant2/1 -> BalCell14_7_Byte_2/1, Integer to Bit Converter1/1
  Selector10/1 -> Bal_11/2
  Integer to Bit Converter15/1 -> [Byte_1_1]
  Bit to Integer Converter5/1 -> BalCell14_7_Byte_4/1
  Selector5/1 -> Bal_6/2
  Selector9/1 -> Bal_10/2
  [Byte_2_2] -> Vector Concatenate7/2
  Constant1/1 -> Bal_12/3, Bal_7/3, Bal_8/3, Bal_9/3, Bal_10/3, Bal_11/3, Bal_1/3, Bal_2/3, Bal_3/3, Bal_4/3, Bal_5/3, Bal_6/3
  Selector8/1 -> Bal_9/2
  Cast To Double/1 -> Vector Concatenate1/2
  Bal_14/1 -> Vector Concatenate/3
  Bal_2/1 -> Vector Concatenate4/2
  Bal_13/1 -> Vector Concatenate/4
  Vector Concatenate7/1 -> MATLAB Function1/1(u_1)
  Bal_Cmd/1 -> Selector11/1, Selector6/1, Selector7/1, Selector8/1, Selector9/1, Selector10/1, Selector/1, Selector1/1, Selector2/1, Selector3/1, Selector4/1, Selector5/1
  MATLAB Function/1(crc) -> Cast To Double/1
  eof_bal/1 -> Vector Concatenate7/6, Vector Concatenate5/2
  bal_on/1 -> Vector Concatenate7/5, Vector Concatenate5/1
  Reshape1/1 -> Bit to Integer Converter5/1
  Vector Concatenate/1 -> [Byte_1_3], Reshape2/1
  [Byte_2_4] -> Vector Concatenate7/4
  Reshape5/1 -> Bit to Integer Converter4/1
  Bal_9/1 -> Vector Concatenate2/2
  Bal_8/1 -> Vector Concatenate2/3
  Noreg_17/1 -> Vector Concatenate/1
  Bal_1/1 -> Vector Concatenate4/3
  Bal_7/1 -> Vector Concatenate2/4
  Vector Concatenate2/1 -> [Byte_1_4], Reshape1/1
  [Byte_1_1] -> Vector Concatenate3/1
  Vector Concatenate4/1 -> [Byte_2_4], Reshape4/1
  Constant5/1 -> Vector Concatenate6/2
  MATLAB Function1/1(crc_1) -> Cast To Double1/1
  Reshape2/1 -> Bit to Integer Converter/1
  Reshape3/1 -> Bit to Integer Converter2/1
  Noreg_2/1 -> Vector Concatenate4/5
  Selector/1 -> Bal_1/2
  Bit to Integer Converter2/1 -> BalCell6_1_Byte_3/1
  Vector Concatenate6/1 -> [Byte2_3], Reshape3/1
  Integer to Bit Converter/1 -> [Byte_2_1]
  Reshape4/1 -> Bit to Integer Converter3/1
  Bal_5/1 -> Vector Concatenate6/4
  Bal_11/1 -> Vector Concatenate3/5, Vector Concatenate1/1
  Reshape/1 -> Bit to Integer Converter1/1
  Constant7/1 -> BalCell6_1_Byte_2/1, Integer to Bit Converter16/1
  [Byte_1_2] -> Vector Concatenate3/2
  Bal_10/1 -> Vector Concatenate2/1
  Bit to Integer Converter3/1 -> BalCell6_1_Byte_4/1
  Constant6/1 -> BalCell6_1_Byte_1/1, Integer to Bit Converter/1
  Bit to Integer Converter4/1 -> BalCell6_1_Byte_5/1
  Selector11/1 -> Bal_12/2
  Bit to Integer Converter1/1 -> BalCell14_7_Byte_5/1
  Noreg_16/1 -> Vector Concatenate/2
  Constant4/1 -> Vector Concatenate6/1
  Integer to Bit Converter16/1 -> [Byte_2_2]
  Vector Concatenate3/1 -> MATLAB Function/1(u)

== stateflow chart BMS_BIL_Wrapper/Test Sequence ==
  state Fly
    State_Required=SRE.Fly
  state step_2
  (default) -> Fly
  Fly -> step_2
  data: State_Required output

== stateflow chart BMS_BIL_Wrapper/BMS_Control/Fault_Severity/Chart ==
  state UV_Fault_Severity
    during:
    if UV_Critical
    Fault_Level.UV = 4;
    elseif UV_Emergency
    Fault_Level.UV = 3;
    elseif UV_PowerLimit
    Fault_Level.UV = 2;
    elseif UV_Warning
    Fault_Level.UV = 1;
    else
    Fault_Level.UV = 0;
    end
  (default) -> UV_Fault_Severity
  data: UV_Warning input boolean; UV_PowerLimit input boolean; UV_Emergency input boolean; UV_Critical input boolean; Fault_Level output Bus: Fault_Level

== stateflow chart BMS_BIL_Wrapper/BMS_Control/Fault_Severity/Chart3 ==
  state UV_Fault_Severity
    during:
    if UT_Critical
    Fault_Level.UT = 4;
    elseif UT_Emergency
    Fault_Level.UT = 3;
    elseif UT_PowerLimit
    Fault_Level.UT = 2;
    elseif UT_Warning
    Fault_Level.UT = 1;
    else
    Fault_Level.UT = 0;
    end
  (default) -> UV_Fault_Severity
  data: UT_Warning input boolean; UT_PowerLimit input boolean; UT_Emergency input boolean; UT_Critical input boolean; Fault_Level output Bus: Fault_Level

== stateflow chart BMS_BIL_Wrapper/BMS_Control/Fault_Severity/Chart1 ==
  state UV_Fault_Severity
    during:
    if OV_Critical
    Fault_Level.OV = 3;
    elseif OV_Stop_Charge
    Fault_Level.OV = 2;
    elseif OV_Warning
    Fault_Level.OV= 1;
    else
    Fault_Level.OV = 0;
    end
  (default) -> UV_Fault_Severity
  data: OV_Warning input boolean; OV_Stop_Charge input boolean; OV_Critical input boolean; Fault_Level output Bus: Fault_Level

== stateflow chart BMS_BIL_Wrapper/BMS_Control/Fault_Severity/Chart2 ==
  state UV_Fault_Severity
    during:
    if OT_Critical
    Fault_Level.OT = 4;
    elseif OT_Emergency
    Fault_Level.OT = 3;
    elseif OT_PowerLimit
    Fault_Level.OT = 2;
    elseif OT_Warning
    Fault_Level.OT = 1;
    else
    Fault_Level.OT = 0;
    end
  (default) -> UV_Fault_Severity
  data: OT_Warning input boolean; OT_PowerLimit input boolean; OT_Emergency input boolean; OT_Critical input boolean; Fault_Level output Bus: Fault_Level

== stateflow chart BMS_BIL_Wrapper/BMS_Control/Subsystem/BMS_States ==
  state Normal_State [parallel]
    settings: executionOrder=1
    state Standby
      en:
      BMS_State_Out= BMS_State.Standbying
    state Charging
      en:
      BMS_State_Out= BMS_State.Charging
    state Flying
      en:
      BMS_State_Out= BMS_State.Flying
    state Fault
      en,du:
      BMS_State_Out= BMS_State.Fault
    (default) -> Standby
    Standby -> Charging [order 2] : [State_Required==SRE.Charge ]
    Standby -> (junction 51) [order 3] : [FaultPresent]
    (junction 51) -> (junction 52)
    Charging -> Standby [order 1] : [(State_Required~=SRE.Charge)...
        | || (State_Required==SRE.Standby) ]
    Standby -> Flying [order 1] : [State_Required== SRE.Fly]
    Flying -> Standby [order 1] : [(State_Required~=SRE.Fly) ||...
        | (State_Required==SRE.Standby) ]
    (junction 43) -> Charging
    Charging -> (junction 41) [order 2]
    Charging -> Fault [order 3] : [FaultPresent]
    Flying -> (junction 43) [order 2] : [State_Required==SRE.Charge]
    (junction 41) -> Flying : [State_Required== SRE.Fly]
    Flying -> Fault [order 3] : [FaultPresent]
    (junction 52) -> Fault
  state Fault_Monitoring [parallel]
    settings: executionOrder=2
    state Monitor_CurrentLim [parallel]
      settings: executionOrder=1
      state No_CurrentLim_Fault
      state Wait
      state OC_Fault
        en:
        FaultPresent=true;
        Fault_out.OC=true;
      (default) -> No_CurrentLim_Fault : {FaultPresent=false;
          |  Fault_out.OC=false;}
      No_CurrentLim_Fault -> Wait : [(Pack_Current< Current_Limits.Discharge_Current_Limit) || ...
          | (Pack_Current> Current_Limits.Charge_Current_Limit)]
      Wait -> No_CurrentLim_Fault [order 2] : [(Pack_Current >= Current_Limits.Discharge_Current_Limit) && ...
          | (Pack_Current <= Current_Limits.Charge_Current_Limit)]
      Wait -> OC_Fault [order 1] : [after(CurrentTimeout, sec)]
    state Monitor_CellVolt [parallel]
      settings: executionOrder=2
      state No_OV_UV
        en,du:
        Delta=abs(V_Batt_Sum-V_Batt_Monitor);
      state OV_Fault
        en:
        FaultPresent=true;
        Fault_out.OV=true;
      state UV_Fault
        en:
        FaultPresent=true;
        Fault_out.UV=true;
      state Sensor_Fault
        en:
        FaultPresent=true;
        Fault_out.VoltSensor=true;
      (default) -> No_OV_UV : {FaultPresent=false;
          | Fault_out.VoltSensor=false;
          | Fault_out.UV=false;
          | Fault_out.OV=false;}
      No_OV_UV -> OV_Fault [order 3] : [Max_Voltage>=Full_Charge_Volt]
      No_OV_UV -> (junction 89) [order 2] : [Min_Voltage <= Cutoff_Volt]
      (junction 89) -> UV_Fault
      No_OV_UV -> Sensor_Fault [order 1] : [Delta>=single(Sensor_Fault_Treshold)]
    state Monitor_CellTemp [parallel]
      settings: executionOrder=3
      state OT_Fault
        en:
        FaultPresent=true;
        Fault_out.OT=true;
      state No_OT_UT
        en, du:
        MaxCellTemp=max(Tmod);
        MinCellTemp=min(Tmod);
      state UT_Fault
        en:
        FaultPresent=true;
        Fault_out.UT=true;
      No_OT_UT -> OT_Fault [order 2] : [MaxCellTemp>=High_TempLim]
      (default) -> No_OT_UT : {FaultPresent=false;
          | Fault_out.OT=false;
          | Fault_out.UT=false;}
      No_OT_UT -> UT_Fault [order 1] : [MinCellTemp<=Low_TempLim]
  data: Current_Limits input Bus: Current_Limits; Tmod input single; Pack_Current input single; V_Batt_Sum input single size=1; State_Required input Enum: SRE; Fault_out output Bus: Fault_out; Max_Voltage input single; Min_Voltage input single; Low_TempLim parameter single; High_TempLim parameter single; Cutoff_Volt parameter single; Full_Charge_Volt parameter single; MaxCellTemp local single; MinCellTemp local single; Delta local single; Sensor_Fault_Treshold parameter double; FaultPresent local boolean; BMS_State_Out output; CurrentTimeout parameter; V_Batt_Monitor input
